simulink model "FIR_lattice"  (R2022b)
settings: Solver=VariableStepAuto  StartTime=0.0  StopTime=10.0  RelTol=1e-3
undefined symbols (not defined in the file): k
libraries: dspsrcs4 x1
settings Model: Creator=adelincraita  LastModifiedBy=crait

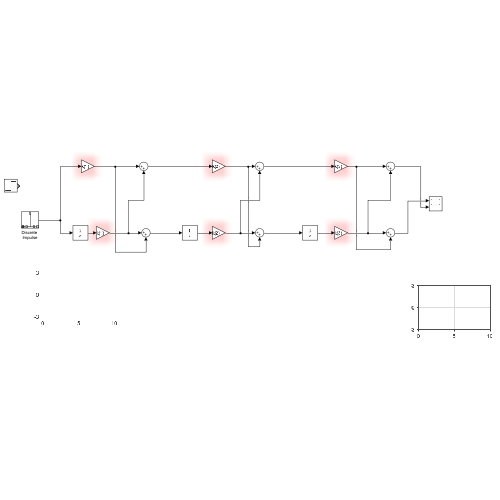
[thumbnail: Simulink's stored preview of the top-level diagram]
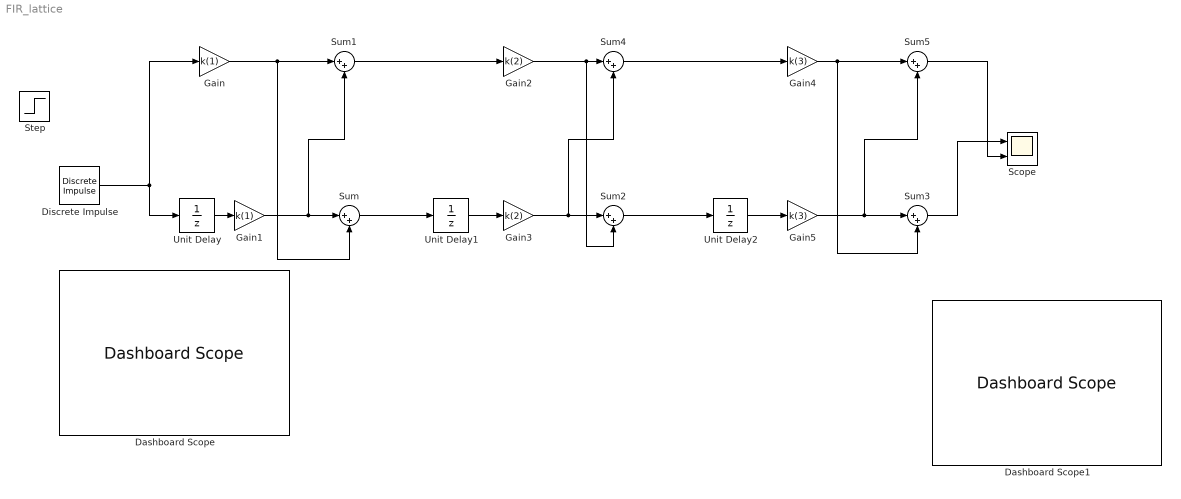
== system FIR_lattice ==
  Dashboard Scope : DashboardScope
  Dashboard Scope1 : DashboardScope
  Discrete Impulse : dspsrcs4/Discrete  Impulse  Delay=0  SampleTime=1  FrameSample=1  OutputFrames=off  dataType=double  isSigned=on  wordLen=16  udDataType=sfix(16)  fracBitsMode=Best precision  numFracBits=15  OutDataTypeStr=double  LastOutDataTypeStr=double
  Gain : Gain  Gain=k(1)
  Gain1 : Gain  Gain=k(1)
  Gain2 : Gain  Gain=k(2)
  Gain3 : Gain  Gain=k(2)
  Gain4 : Gain  Gain=k(3)
  Gain5 : Gain  Gain=k(3)
  Scope : Scope  NumInputPorts=2
  Step : Step  SampleTime=0
  Sum{,1..5} (6 alike) : Sum  Inputs=|++
  Unit Delay : UnitDelay  SampleTime=-1  HasFrameUpgradeWarning=on
  Unit Delay1 : UnitDelay  SampleTime=-1  HasFrameUpgradeWarning=on
  Unit Delay2 : UnitDelay  SampleTime=-1  HasFrameUpgradeWarning=on
  wires:
  Unit Delay/1 -> Gain1/1
  Sum/1 -> Unit Delay1/1
  Unit Delay1/1 -> Gain3/1
  Sum2/1 -> Unit Delay2/1
  Unit Delay2/1 -> Gain5/1
  Sum1/1 -> Gain2/1
  Gain/1 -> Sum/2, Sum1/1
  Gain1/1 -> Sum1/2, Sum/1
  Gain2/1 -> Sum2/2, Sum4/1
  Gain3/1 -> Sum4/2, Sum2/1
  Sum4/1 -> Gain4/1
  Gain5/1 -> Sum5/2, Sum3/1
  Gain4/1 -> Sum3/2, Sum5/1
  Sum3/1 -> Scope/1
  Sum5/1 -> Scope/2
  Discrete Impulse/1 -> Gain/1, Unit Delay/1
